simulink model "OFDMA_Analogico"  (R2018a)
settings: Solver=FixedStepAuto  StartTime=0.0  StopTime=M*CantBit  FixedStep=Tsampling  RelTol=1e-3
values from neighbouring files (symbols this model uses):
  CantMPerSimbOFDM = round(TsOFDM/Tsampling)    [OFDMA_analogico.m]
  EsOFDM = 2    [OFDMA_analogico.m]
  F1 = FsepOFDM*2    [OFDMA_analogico.m]
  F2 = FsepOFDM*3    [OFDMA_analogico.m]
  F3 = FsepOFDM*4    [OFDMA_analogico.m]
  F4 = FsepOFDM*5    [OFDMA_analogico.m]
  Tb3 = 1/Rb3    (= 0.0005)    [OFDMA_analogico.m]
  Tb4 = 1/Rb4    (= 0.000333333333333)    [OFDMA_analogico.m]
  Ts1 = Tb1    (= 0.001)    [OFDMA_analogico.m]
  Ts2 = Tb2    (= 0.001)    [OFDMA_analogico.m]
  Ts3 = 2*Tb3    (= 0.001)    [OFDMA_analogico.m]
  Ts4 = 3*Tb4    (= 0.001)    [OFDMA_analogico.m]
  Tsampling = M/N    [OFDMA_analogico.m]
libraries: commdigbbndpm3 x8, dspsigops x8, commrandsrc3 x4
settings Model: Creator=lukit  LastModifiedBy=geroo
settings DebuggingCC: LibraryContextMissingDiagnostic=warning
settings SFSimCC: SimUseLocalCustomCode=on
settings RTWCC: RTWUseLocalCustomCode=on

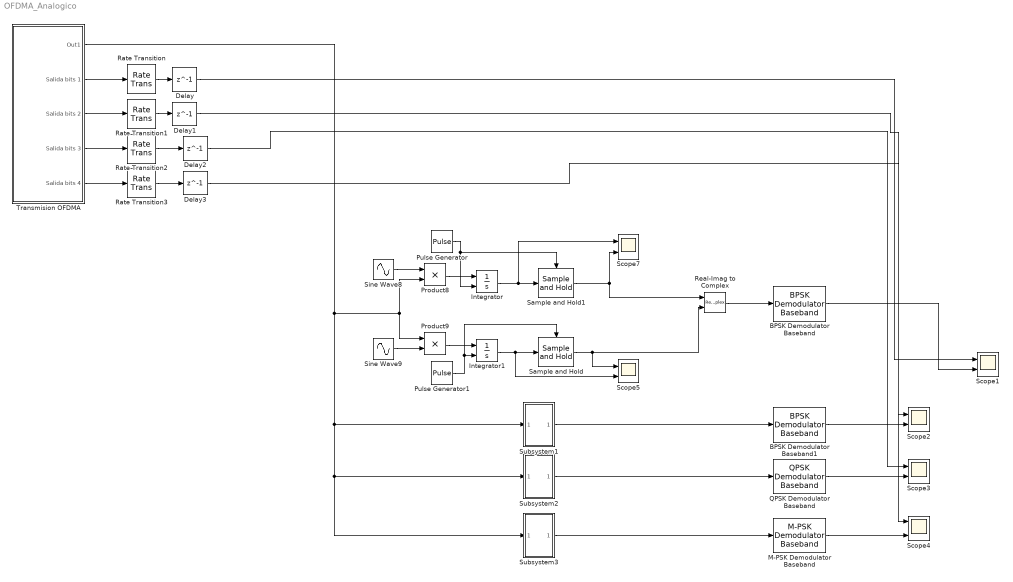
== system OFDMA_Analogico ==
  BPSK Demodulator Baseband : commdigbbndpm3/BPSK Demodulator Baseband  DecType=Hard decision  VarSource=Dialog  Variance=1  Ph=0  outDtype=Inherit via internal rule  derotateFactorWordLen=16  derotateFactorDataTypeStr=Inherit: Same word length as input  derotateFactorLastDataTypeStr=Inherit: Same word length as input
  BPSK Demodulator Baseband1 : commdigbbndpm3/BPSK Demodulator Baseband  DecType=Hard decision  VarSource=Dialog  Variance=1  Ph=0  outDtype=Inherit via internal rule  derotateFactorWordLen=16  derotateFactorDataTypeStr=Inherit: Same word length as input  derotateFactorLastDataTypeStr=Inherit: Same word length as input
  Delay : Delay  DelayLength=1  InitialCondition=0  InputProcessing=Columns as channels (frame based)  SampleTime=Ts1
  Delay1 : Delay  DelayLength=1  InitialCondition=0  InputProcessing=Columns as channels (frame based)  SampleTime=Ts2
  Delay2 : Delay  DelayLength=1  InitialCondition=0  InputProcessing=Columns as channels (frame based)  SampleTime=Ts3
  Delay3 : Delay  DelayLength=1  InitialCondition=0  InputProcessing=Columns as channels (frame based)  SampleTime=Ts4
  Integrator : Integrator  ExternalReset=rising
  Integrator1 : Integrator  ExternalReset=rising
  M-PSK Demodulator Baseband : commdigbbndpm3/M-PSK Demodulator Baseband  M=8  OutType=Integer  DecType=Hard decision  VarSource=Dialog  Variance=1  Dec=Gray  Mapping=[0:7]  Ph=0  outDtype1=Inherit via internal rule  outDtype2=Inherit via internal rule  derotateFactorWordLen=16  derotateFactorDataTypeStr=Inherit: Same word length as input  derotateFactorLastDataTypeStr=Inherit: Same word length as input
      settings: SourceProductName=Communications System Toolbox
  Product8 : Product
  Product9 : Product
  Pulse Generator : DiscretePulseGenerator  PulseType=Time based  Period=Ts1  PulseWidth=99.9
  Pulse Generator1 : DiscretePulseGenerator  PulseType=Time based  Period=Ts1  PulseWidth=99.9
  QPSK Demodulator Baseband : commdigbbndpm3/QPSK Demodulator Baseband  OutType=Integer  DecType=Hard decision  VarSource=Dialog  Variance=1  Dec=Gray  Ph=0  outDtype1=Inherit via internal rule  outDtype2=Inherit via internal rule  derotateFactorWordLen=16  derotateFactorDataTypeStr=Inherit: Same word length as input  derotateFactorLastDataTypeStr=Inherit: Same word length as input
  Rate Transition : RateTransition  OutPortSampleTime=Ts1
  Rate Transition1 : RateTransition  OutPortSampleTime=Ts2
  Rate Transition2 : RateTransition  OutPortSampleTime=Tsampling
  Rate Transition3 : RateTransition  OutPortSampleTime=Tsampling
  Real-Imag to Complex : RealImagToComplex
  Sample and Hold : dspsigops/Sample and Hold  trig=Falling edge  initCond=0  latchinput=off
  Sample and Hold1 : dspsigops/Sample and Hold  trig=Falling edge  initCond=0  latchinput=off
  Scope{1..5,7} (6 alike) : Scope  NumInputPorts=2
  Sine Wave8 : Sin  Amplitude=sqrt(2/Ts1)  Frequency=2*pi*F1  Phase=pi/2  SampleTime=Tsampling
  Sine Wave9 : Sin  Amplitude=sqrt(2/Ts1)  Frequency=2*pi*F1  SampleTime=Tsampling
  Subsystem1 : Subsystem
  Subsystem2 : Subsystem
  Subsystem3 : Subsystem
  Transmision OFDMA : Subsystem
  wires:
  BPSK Demodulator Baseband/1 -> Scope1/2
  Transmision OFDMA/2(Salida bits 1) -> Rate Transition/1
  Delay/1 -> Scope1/1
  Rate Transition/1 -> Delay/1
  Real-Imag to Complex/1 -> BPSK Demodulator Baseband/1
  Subsystem1/1(Out1) -> BPSK Demodulator Baseband1/1
  Subsystem2/1(Out1) -> QPSK Demodulator Baseband/1
  Subsystem3/1(Out1) -> M-PSK Demodulator Baseband/1
  QPSK Demodulator Baseband/1 -> Scope3/2
  BPSK Demodulator Baseband1/1 -> Scope2/2
  Rate Transition1/1 -> Delay1/1
  Rate Transition3/1 -> Delay3/1
  Transmision OFDMA/3(Salida bits 2) -> Rate Transition1/1
  Delay1/1 -> Scope2/1
  Transmision OFDMA/5(Salida bits 4) -> Rate Transition3/1
  Delay3/1 -> Scope4/1
  Rate Transition2/1 -> Delay2/1
  Transmision OFDMA/4(Salida bits 3) -> Rate Transition2/1
  Delay2/1 -> Scope3/1
  M-PSK Demodulator Baseband/1 -> Scope4/2
  Transmision OFDMA/1(Out1) -> Product8/2, Product9/1, Subsystem3/1(In1), Subsystem2/1(In1), Subsystem1/1(In1)
  Integrator1/1 -> Scope5/2, Sample and Hold/1
  Integrator/1 -> Scope7/1, Sample and Hold1/1
  Pulse Generator/1 -> Integrator/2, Sample and Hold1/Trigger
  Sine Wave8/1 -> Product8/1
  Pulse Generator1/1 -> Integrator1/2, Sample and Hold/Trigger
  Sample and Hold1/1 -> Scope7/2, Real-Imag to Complex/1
  Sine Wave9/1 -> Product9/2
  Product8/1 -> Integrator/1
  Product9/1 -> Integrator1/1
  Sample and Hold/1 -> Real-Imag to Complex/2, Scope5/1

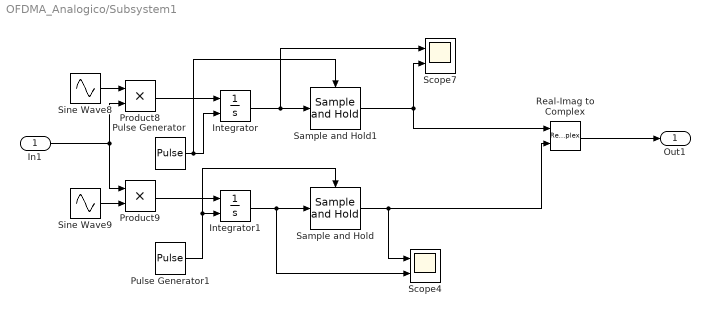
== system OFDMA_Analogico/Subsystem1 ==
  In1 : Inport
  Integrator : Integrator  ExternalReset=rising
  Integrator1 : Integrator  ExternalReset=rising
  Product8 : Product
  Product9 : Product
  Pulse Generator : DiscretePulseGenerator  PulseType=Time based  Period=Ts2  PulseWidth=99.9
  Pulse Generator1 : DiscretePulseGenerator  PulseType=Time based  Period=Ts2  PulseWidth=99.9
  Real-Imag to Complex : RealImagToComplex
  Sample and Hold : dspsigops/Sample and Hold  trig=Falling edge  initCond=0  latchinput=off
  Sample and Hold1 : dspsigops/Sample and Hold  trig=Falling edge  initCond=0  latchinput=off
  Scope4 : Scope  NumInputPorts=2
  Scope7 : Scope  NumInputPorts=2
  Sine Wave8 : Sin  Amplitude=sqrt(2/Ts2)  Frequency=2*pi*F2  Phase=pi/2  SampleTime=Tsampling
  Sine Wave9 : Sin  Amplitude=sqrt(2/Ts1)  Frequency=2*pi*F1  SampleTime=Tsampling
  Out1 : Outport
  wires:
  Product8/1 -> Integrator/1
  Integrator1/1 -> Scope4/2, Sample and Hold/1
  Product9/1 -> Integrator1/1
  Real-Imag to Complex/1 -> Out1/1
  Sine Wave8/1 -> Product8/1
  Sample and Hold/1 -> Real-Imag to Complex/2, Scope4/1
  Pulse Generator/1 -> Integrator/2, Sample and Hold1/Trigger
  Sample and Hold1/1 -> Scope7/2, Real-Imag to Complex/1
  Pulse Generator1/1 -> Integrator1/2, Sample and Hold/Trigger
  Sine Wave9/1 -> Product9/2
  Integrator/1 -> Scope7/1, Sample and Hold1/1
  In1/1 -> Product8/2, Product9/1

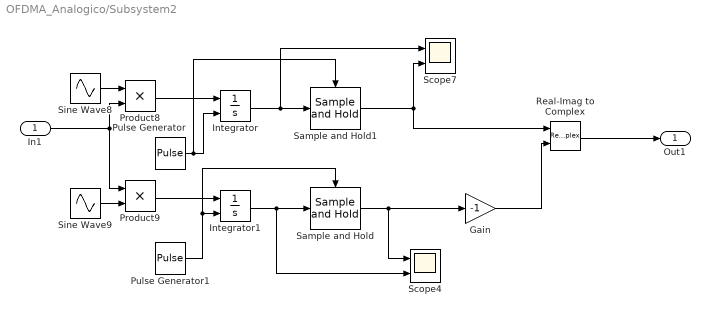
== system OFDMA_Analogico/Subsystem2 ==
  In1 : Inport
  Gain : Gain  Gain=-1
  Integrator : Integrator  ExternalReset=rising
  Integrator1 : Integrator  ExternalReset=rising
  Product8 : Product
  Product9 : Product
  Pulse Generator : DiscretePulseGenerator  PulseType=Time based  Period=Ts3  PulseWidth=99.9
  Pulse Generator1 : DiscretePulseGenerator  PulseType=Time based  Period=Ts3  PulseWidth=99.9
  Real-Imag to Complex : RealImagToComplex
  Sample and Hold : dspsigops/Sample and Hold  trig=Falling edge  initCond=0  latchinput=off
  Sample and Hold1 : dspsigops/Sample and Hold  trig=Falling edge  initCond=0  latchinput=off
  Scope4 : Scope  NumInputPorts=2
  Scope7 : Scope  NumInputPorts=2
  Sine Wave8 : Sin  Amplitude=sqrt(2/Ts3)  Frequency=2*pi*F3  Phase=pi/2  SampleTime=Tsampling
  Sine Wave9 : Sin  Amplitude=sqrt(2/Ts3)  Frequency=2*pi*F3  SampleTime=Tsampling
  Out1 : Outport
  wires:
  Product8/1 -> Integrator/1
  Integrator1/1 -> Scope4/2, Sample and Hold/1
  Product9/1 -> Integrator1/1
  Real-Imag to Complex/1 -> Out1/1
  Sine Wave8/1 -> Product8/1
  Sample and Hold/1 -> Gain/1, Scope4/1
  Pulse Generator/1 -> Integrator/2, Sample and Hold1/Trigger
  Sample and Hold1/1 -> Scope7/2, Real-Imag to Complex/1
  Pulse Generator1/1 -> Integrator1/2, Sample and Hold/Trigger
  Sine Wave9/1 -> Product9/2
  Integrator/1 -> Scope7/1, Sample and Hold1/1
  In1/1 -> Product9/1, Product8/2
  Gain/1 -> Real-Imag to Complex/2

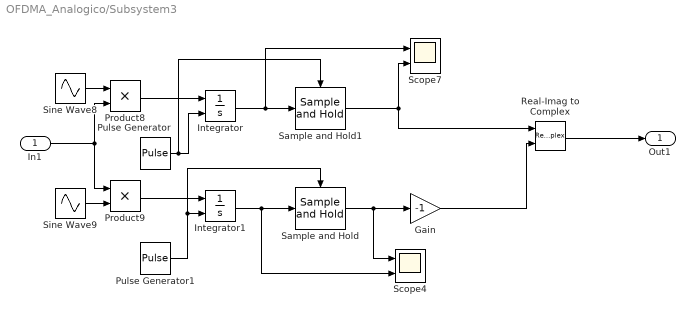
== system OFDMA_Analogico/Subsystem3 ==
  In1 : Inport
  Gain : Gain  Gain=-1
  Integrator : Integrator  ExternalReset=rising
  Integrator1 : Integrator  ExternalReset=rising
  Product8 : Product
  Product9 : Product
  Pulse Generator : DiscretePulseGenerator  PulseType=Time based  Period=Ts4  PulseWidth=99.9
  Pulse Generator1 : DiscretePulseGenerator  PulseType=Time based  Period=Ts4  PulseWidth=99.9
  Real-Imag to Complex : RealImagToComplex
  Sample and Hold : dspsigops/Sample and Hold  trig=Falling edge  initCond=0  latchinput=off
  Sample and Hold1 : dspsigops/Sample and Hold  trig=Falling edge  initCond=0  latchinput=off
  Scope4 : Scope  NumInputPorts=2
  Scope7 : Scope  NumInputPorts=2
  Sine Wave8 : Sin  Amplitude=sqrt(2/Ts4)  Frequency=2*pi*F4  Phase=pi/2  SampleTime=Tsampling
  Sine Wave9 : Sin  Amplitude=sqrt(2/Ts4)  Frequency=2*pi*F4  SampleTime=Tsampling
  Out1 : Outport
  wires:
  Product8/1 -> Integrator/1
  Integrator1/1 -> Scope4/2, Sample and Hold/1
  Product9/1 -> Integrator1/1
  Real-Imag to Complex/1 -> Out1/1
  Sine Wave8/1 -> Product8/1
  Sample and Hold/1 -> Gain/1, Scope4/1
  Pulse Generator/1 -> Integrator/2, Sample and Hold1/Trigger
  Sample and Hold1/1 -> Scope7/2, Real-Imag to Complex/1
  Pulse Generator1/1 -> Integrator1/2, Sample and Hold/Trigger
  Sine Wave9/1 -> Product9/2
  Integrator/1 -> Scope7/1, Sample and Hold1/1
  In1/1 -> Product8/2, Product9/1
  Gain/1 -> Real-Imag to Complex/2

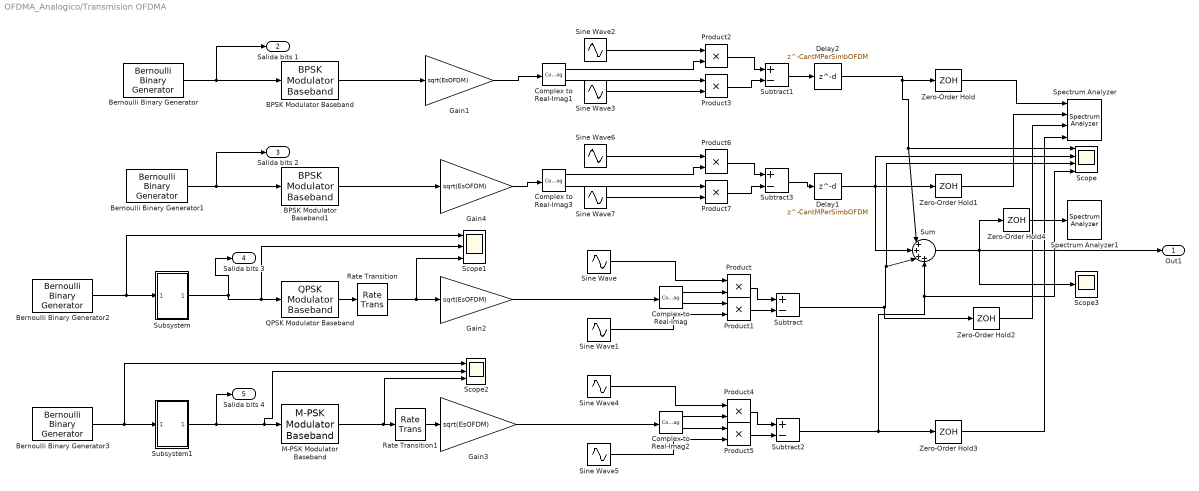
== system OFDMA_Analogico/Transmision OFDMA ==
  BPSK Modulator Baseband : commdigbbndpm3/BPSK Modulator Baseband  Ph=0  outDtype=double  outWordLen=16  outUDDataType=sfix(16)  outFracLenMode=Best precision  outFracLen=15  outDataTypeStr=double  outLastDataTypeStr=double
  BPSK Modulator Baseband1 : commdigbbndpm3/BPSK Modulator Baseband  Ph=0  outDtype=double  outWordLen=16  outUDDataType=sfix(16)  outFracLenMode=Best precision  outFracLen=15  outDataTypeStr=double  outLastDataTypeStr=double
  Bernoulli Binary Generator : commrandsrc3/Bernoulli Binary Generator  ProbabilityOfZero=0.5  SeedSource=Auto  Seed=0  SampleTime=Ts1  SamplesPerFrame=1  OutputDataType=double  SimulateUsing=Interpreted execution
  Bernoulli Binary Generator1 : commrandsrc3/Bernoulli Binary Generator  ProbabilityOfZero=0.5  SeedSource=Auto  Seed=0  SampleTime=Ts2  SamplesPerFrame=1  OutputDataType=double  SimulateUsing=Interpreted execution
  Bernoulli Binary Generator2 : commrandsrc3/Bernoulli Binary Generator  ProbabilityOfZero=0.5  SeedSource=Auto  Seed=0  SampleTime=Tb3  SamplesPerFrame=1  OutputDataType=double  SimulateUsing=Interpreted execution
  Bernoulli Binary Generator3 : commrandsrc3/Bernoulli Binary Generator  ProbabilityOfZero=0.5  SeedSource=Auto  Seed=0  SampleTime=Tb4  SamplesPerFrame=1  OutputDataType=double  SimulateUsing=Interpreted execution
  Complex to Real-Imag{,1..3} (4 alike) : ComplexToRealImag
  Delay1 : Delay  DelayLength=CantMPerSimbOFDM  InitialCondition=0  SampleTime=Tsampling
  Delay2 : Delay  DelayLength=CantMPerSimbOFDM  InitialCondition=0  SampleTime=Tsampling
  Gain{1..4} (4 alike) : Gain  Gain=sqrt(EsOFDM)
  M-PSK Modulator Baseband : commdigbbndpm3/M-PSK Modulator Baseband  M=8  InType=Integer  Enc=Gray  Mapping=[0:7]  Ph=0  outDtype=double  outWordLen=16  outUDDataType=sfix(16)  outFracLenMode=Best precision  outFracLen=15  outDataTypeStr=double  outLastDataTypeStr=double
      settings: SourceProductName=Communications System Toolbox
  Product{,1..7} (8 alike) : Product
  QPSK Modulator Baseband : commdigbbndpm3/QPSK Modulator Baseband  InType=Integer  Enc=Gray  Ph=0  outDtype=double  outWordLen=16  outUDDataType=sfix(16)  outFracLenMode=Best precision  outFracLen=15  outDataTypeStr=double  outLastDataTypeStr=double
  Rate Transition : RateTransition  OutPortSampleTime=Tsampling
  Rate Transition1 : RateTransition  OutPortSampleTime=Tsampling
  Scope : Scope  NumInputPorts=4
  Scope1 : Scope  NumInputPorts=3
  Scope2 : Scope  NumInputPorts=3
  Scope3 : Scope
  Sine Wave : Sin  Amplitude=sqrt(2/Ts3)  Frequency=2*pi*F3  Phase=pi/2  SampleTime=Tsampling
  Sine Wave1 : Sin  Amplitude=sqrt(2/Ts3)  Frequency=2*pi*F3  SampleTime=Tsampling
  Sine Wave2 : Sin  Amplitude=sqrt(2/Ts1)  Frequency=2*pi*F1  Phase=pi/2  SampleTime=Tsampling
  Sine Wave3 : Sin  Amplitude=sqrt(2/Ts1)  Frequency=2*pi*F1  SampleTime=Tsampling
  Sine Wave4 : Sin  Amplitude=sqrt(2/Ts4)  Frequency=2*pi*F4  Phase=pi/2  SampleTime=Tsampling
  Sine Wave5 : Sin  Amplitude=sqrt(2/Ts4)  Frequency=2*pi*F4  SampleTime=Tsampling
  Sine Wave6 : Sin  Amplitude=sqrt(2/Ts2)  Frequency=2*pi*F2  Phase=pi/2  SampleTime=Tsampling
  Sine Wave7 : Sin  Amplitude=sqrt(2/Ts2)  Frequency=2*pi*F2  SampleTime=Tsampling
  Spectrum Analyzer : SpectrumAnalyzer  NumInputPorts=4
  Spectrum Analyzer1 : SpectrumAnalyzer
  Subsystem : Subsystem
  Subsystem1 : Subsystem
  Subtract{,1..3} (4 alike) : Sum  Inputs=+-
  Sum : Sum  Inputs=|++++
  Zero-Order Hold{,1..4} (5 alike) : ZeroOrderHold  SampleTime=-1
  Out1 : Outport
  Salida bits 1 : Outport  Port=2
  Salida bits 2 : Outport  Port=3
  Salida bits 3 : Outport  Port=4
  Salida bits 4 : Outport  Port=5
  wires:
  Product3/1 -> Subtract1/2
  Zero-Order Hold/1 -> Spectrum Analyzer/1
  Subtract3/1 -> Delay1/1
  Subtract2/1 -> Zero-Order Hold3/1, Scope/4, Sum/4
  Complex to Real-Imag3/1 -> Product6/2
  Gain2/1 -> Complex to Real-Imag/1
  Sine Wave2/1 -> Product2/1
  Product2/1 -> Subtract1/1
  Complex to Real-Imag1/2 -> Product3/1
  Gain3/1 -> Complex to Real-Imag2/1
  Bernoulli Binary Generator1/1 -> Salida bits 2/1, BPSK Modulator Baseband1/1
  QPSK Modulator Baseband/1 -> Rate Transition/1
  Complex to Real-Imag/1 -> Product/2
  M-PSK Modulator Baseband/1 -> Scope2/3, Rate Transition1/1
  Sine Wave5/1 -> Product5/2
  Product6/1 -> Subtract3/1
  Product5/1 -> Subtract2/2
  Complex to Real-Imag1/1 -> Product2/2
  Sine Wave6/1 -> Product6/1
  Product1/1 -> Subtract/2
  Sine Wave/1 -> Product/1
  Zero-Order Hold4/1 -> Spectrum Analyzer1/1
  BPSK Modulator Baseband/1 -> Gain1/1
  Sine Wave3/1 -> Product3/2
  Subtract/1 -> Zero-Order Hold2/1, Scope/3, Sum/3
  Product/1 -> Subtract/1
  Complex to Real-Imag2/2 -> Product5/1
  Sine Wave7/1 -> Product7/2
  Bernoulli Binary Generator3/1 -> Scope2/1, Subsystem1/1(In1)
  Complex to Real-Imag2/1 -> Product4/2
  Product7/1 -> Subtract3/2
  BPSK Modulator Baseband1/1 -> Gain4/1
  Complex to Real-Imag/2 -> Product1/1
  Product4/1 -> Subtract2/1
  Complex to Real-Imag3/2 -> Product7/1
  Sum/1 -> Out1/1, Zero-Order Hold4/1, Scope3/1
  Zero-Order Hold2/1 -> Spectrum Analyzer/3
  Gain4/1 -> Complex to Real-Imag3/1
  Gain1/1 -> Complex to Real-Imag1/1
  Sine Wave4/1 -> Product4/1
  Zero-Order Hold1/1 -> Spectrum Analyzer/2
  Zero-Order Hold3/1 -> Spectrum Analyzer/4
  Sine Wave1/1 -> Product1/2
  Bernoulli Binary Generator/1 -> BPSK Modulator Baseband/1, Salida bits 1/1
  Bernoulli Binary Generator2/1 -> Subsystem/1(In1), Scope1/1
  Subsystem/1(Out1) -> Scope1/2, QPSK Modulator Baseband/1, Salida bits 3/1
  Subsystem1/1(Out1) -> Salida bits 4/1, Scope2/2, M-PSK Modulator Baseband/1
  Rate Transition/1 -> Scope1/3, Gain2/1
  Rate Transition1/1 -> Gain3/1
  Subtract1/1 -> Delay2/1
  Delay1/1 -> Zero-Order Hold1/1, Sum/2, Scope/2
  Delay2/1 -> Scope/1, Sum/1, Zero-Order Hold/1

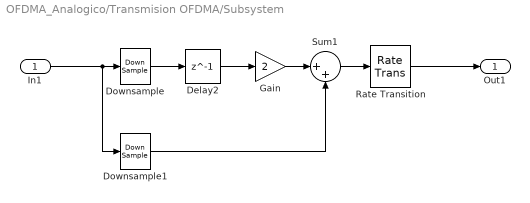
== system OFDMA_Analogico/Transmision OFDMA/Subsystem ==
  In1 : Inport
  Delay2 : Delay  DelayLength=1  InitialCondition=0
  Downsample : DownSample  RateOptions=Allow multirate processing
  Downsample1 : DownSample  phase=1  RateOptions=Allow multirate processing
  Gain : Gain  Gain=2
  Rate Transition : RateTransition  OutPortSampleTime=Ts3
  Sum1 : Sum  Inputs=|++
  Out1 : Outport
  wires:
  Gain/1 -> Sum1/1
  Downsample/1 -> Delay2/1
  Downsample1/1 -> Sum1/2
  Rate Transition/1 -> Out1/1
  Delay2/1 -> Gain/1
  In1/1 -> Downsample1/1, Downsample/1
  Sum1/1 -> Rate Transition/1

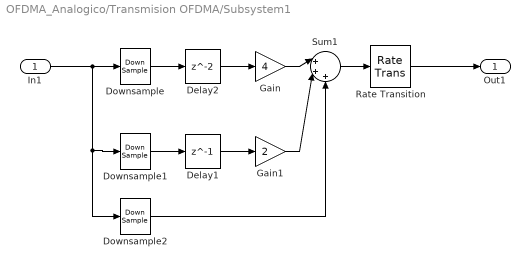
== system OFDMA_Analogico/Transmision OFDMA/Subsystem1 ==
  In1 : Inport
  Delay1 : Delay  DelayLength=1  InitialCondition=0
  Delay2 : Delay  InitialCondition=0
  Downsample : DownSample  N=3  RateOptions=Allow multirate processing
  Downsample1 : DownSample  N=3  phase=1  RateOptions=Allow multirate processing
  Downsample2 : DownSample  N=3  phase=2  RateOptions=Allow multirate processing
  Gain : Gain  Gain=4
  Gain1 : Gain  Gain=2
  Rate Transition : RateTransition  OutPortSampleTime=Ts4
  Sum1 : Sum  Inputs=|+++
  Out1 : Outport
  wires:
  Gain/1 -> Sum1/1
  Downsample/1 -> Delay2/1
  Downsample1/1 -> Delay1/1
  Rate Transition/1 -> Out1/1
  Delay2/1 -> Gain/1
  In1/1 -> Downsample/1, Downsample1/1, Downsample2/1
  Sum1/1 -> Rate Transition/1
  Downsample2/1 -> Sum1/3
  Gain1/1 -> Sum1/2
  Delay1/1 -> Gain1/1
